simulink model "tarcie"  (R2018b)
settings: Solver=ode4  StartTime=0.0  StopTime=10.0  FixedStep=0.1  RelTol=1e-3
values from neighbouring files (symbols this model uses):
  a = 0.9    [dane.m]    (also in untitled.m)
  b = 1.07    [dane.m]    (also in untitled.m)
  c = 0.2773    [dane.m]    (also in untitled.m)
  d = 0.0026    [dane.m]    (also in untitled.m)
settings Model: Creator=lpa1  LastModifiedBy=lpa1

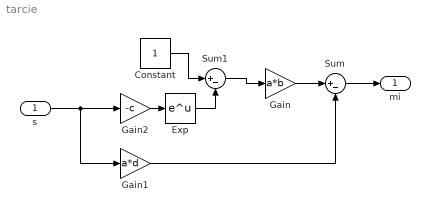
== system tarcie ==
  s : Inport  OutMin=0  OutMax=1
  Constant : Constant
  Exp : Math  SaturateOnIntegerOverflow=on
  Gain : Gain  Gain=a*b
  Gain1 : Gain  Gain=a*d
  Gain2 : Gain  Gain=-c
  Sum : Sum  Inputs=|+-
  Sum1 : Sum  Inputs=|+-
  "mi " : Outport  OutMin=0  OutMax=1
  wires:
  Gain1/1 -> Sum/2
  Sum1/1 -> Gain/1
  Exp/1 -> Sum1/2
  Gain2/1 -> Exp/1
  Constant/1 -> Sum1/1
  Gain/1 -> Sum/1
  Sum/1 -> "mi "/1
  s/1 -> Gain1/1, Gain2/1
